simulink model "InvertedPendulum"  (R2015b)
settings: Solver=FixedStepAuto  StartTime=0.0  StopTime=simtime  FixedStep=1/30  RelTol=1e-3
values from neighbouring files (symbols this model uses):
  b = 0.01    [inverted_pendulum.m]    (also in inverted_pendulum_controlled.m)
  d = 0.02    [inverted_pendulum.m]    (also in inverted_pendulum_controlled.m)
  F1 = 5    [inverted_pendulum.m]
  F1_time = 3    [inverted_pendulum.m]
  F2 = 0    [inverted_pendulum.m]    (also in inverted_pendulum_controlled.m = -1)
  F2_time = 0    [inverted_pendulum.m]    (also in inverted_pendulum_controlled.m = 4)
  g = 9.82    [inverted_pendulum.m]    (also in inverted_pendulum_controlled.m)
  l = 0.3    [inverted_pendulum.m]    (also in inverted_pendulum_controlled.m)
  m = 0.2    [inverted_pendulum.m]    (also in inverted_pendulum_controlled.m)
  M = 0.5    [inverted_pendulum.m]    (also in inverted_pendulum_controlled.m)
  theta_init = pi/6    (= 0.523598775598)    [inverted_pendulum.m]    (also in inverted_pendulum_controlled.m = 0.2)
settings Model: Creator=Andreas  LastModifiedBy=Andreas

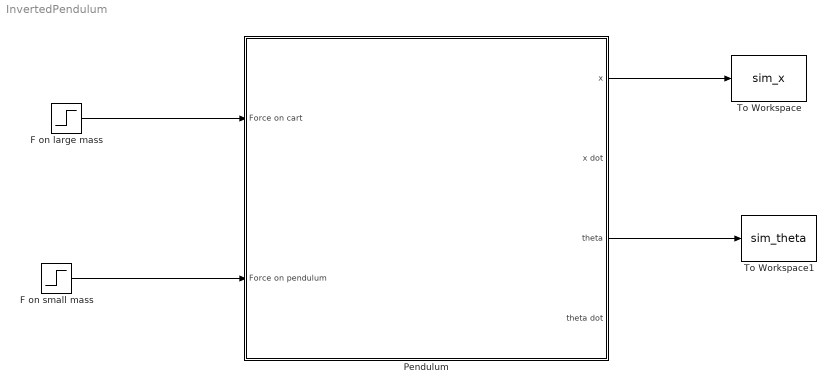
== system InvertedPendulum ==
  F on large mass : Step  Time=F1_time  After=F1  SampleTime=0
  F on small mass : Step  Time=F2_time  After=F2  SampleTime=0
  Pendulum : Subsystem
      mask Display:
      | image('invpend.jpg')
      | port_label('input', 1, 'Force on cart')
      | port_label('input', 2, 'Force on pendulum')
      | port_label('output', 1, 'x')
      | port_label('output', 2, 'x dot')
      | port_label('output', 3, 'theta')
      | port_label('output', 4, 'theta dot')
  To Workspace : ToWorkspace  VariableName=sim_x  SaveFormat=Timeseries  SampleTime=-1
  To Workspace1 : ToWorkspace  VariableName=sim_theta  SaveFormat=Timeseries  SampleTime=-1
  wires:
  F on small mass/1 -> Pendulum/2(Force on pendulum)
  Pendulum/3(theta) -> To Workspace1/1
  Pendulum/1("x ") -> To Workspace/1
  F on large mass/1 -> Pendulum/1(Force on cart)

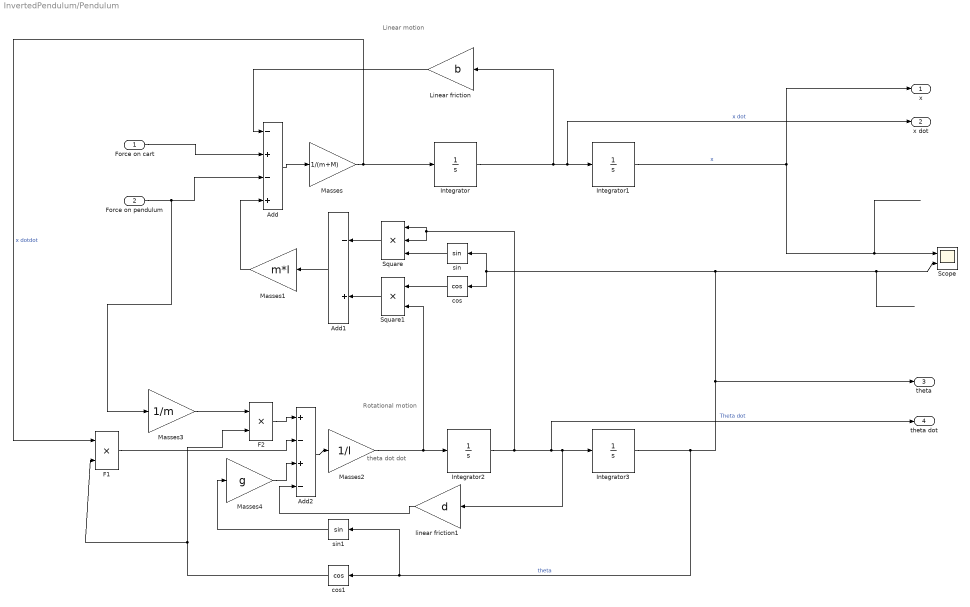
== system InvertedPendulum/Pendulum ==
  note: theta dot dot
  note: Linear motion
  note: Rotational motion
  Force on cart : Inport
  Force on pendulum : Inport  Port=2
  Add : Sum  Inputs=-+-+
  Add1 : Sum  Inputs=-+
  Add2 : Sum  Inputs=+-+-
  F1 : Product
  F2 : Product
  Integrator : Integrator
  Integrator1 : Integrator
  Integrator2 : Integrator
  Integrator3 : Integrator  InitialCondition=theta_init
  Linear friction : Gain  Gain=b
  Masses : Gain  Gain=1/(m+M)
  Masses1 : Gain  Gain=m*l
  Masses2 : Gain  Gain=1/l
  Masses3 : Gain  Gain=1/m
  Masses4 : Gain  Gain=g
  Scope : Scope  NumInputPorts=2
  Square : Product  Inputs=3
  Square1 : Product
  cos : Trigonometry  Operator=cos
  cos1 : Trigonometry  Operator=cos
  linear friction1 : Gain  Gain=d
  sin : Trigonometry
  sin1 : Trigonometry
  "x " : Outport
  x dot : Outport  Port=2
  theta : Outport  Port=3
  theta dot : Outport  Port=4
  wires:
  Force on pendulum/1 -> Add/3, Masses3/1
  Integrator1/1 -> Scope/1, "x "/1  "x"
  linear friction1/1 -> Add2/4
  Force on cart/1 -> Add/2
  Masses/1 -> F1/1, Integrator/1  "x dotdot"
  Add/1 -> Masses/1
  F2/1 -> Add2/1
  F1/1 -> Add2/2
  Integrator3/1 -> sin1/1, cos1/1, Scope/2, cos/1, sin/1, theta/1  "theta"
  cos1/1 -> F2/2, F1/2
  Linear friction/1 -> Add/1
  Add1/1 -> Masses1/1
  Square1/1 -> Add1/2
  Masses1/1 -> Add/4
  sin/1 -> Square/3
  Integrator2/1 -> Square/2, Square/1, theta dot/1, linear friction1/1, Integrator3/1  "Theta dot"
  Masses2/1 -> Square1/2, Integrator2/1
  Integrator/1 -> Linear friction/1, x dot/1, Integrator1/1  "x dot"
  Add2/1 -> Masses2/1
  Masses3/1 -> F2/1
  Square/1 -> Add1/1
  sin1/1 -> Masses4/1
  Masses4/1 -> Add2/3
  cos/1 -> Square1/1
